simulink model "DKM"  (R2015a)
settings: Solver=ode45  StartTime=0.0  StopTime=10.0  RelTol=1e-3
values from neighbouring files (symbols this model uses):
  L = 0.13    [staticInit.m]
  r = 0.1    [staticInit.m]
settings Model: CovModelRefEnable=off  Creator=Subodh  LastModifiedBy=Subodh
settings DataIOCC: SaveFormat=Dataset
settings HardwareCC: ProdBitPerPointer=64  ProdLargestAtomicFloat=Float  ProdIntDivRoundTo=Zero  ProdEndianess=LittleEndian  ProdHWDeviceType=Specified
settings GRTTargetCC: GeneratePreprocessorConditionals=Use local settings

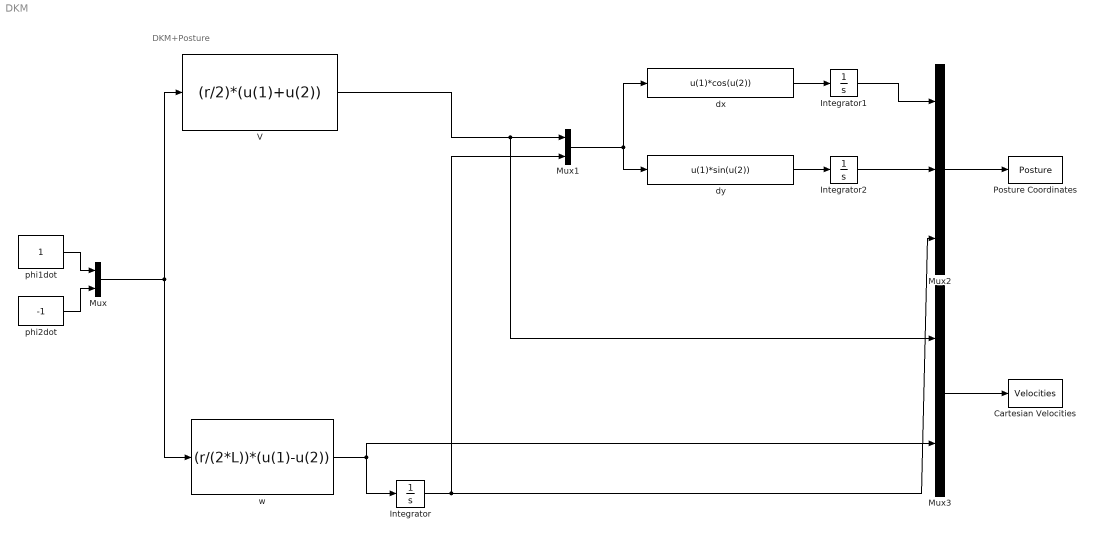
== system DKM ==
  note: DKM+Posture
  Cartesian Velocities : ToWorkspace  VariableName=Velocities  SampleTime=-1
  Integrator : Integrator  InitialCondition=pi
  Integrator1 : Integrator  InitialCondition=2.45
  Integrator2 : Integrator
  Mux : Mux  Inputs=2
  Mux1 : Mux  Inputs=2
  Mux2 : Mux  Inputs=3
  Mux3 : Mux  Inputs=2
  Posture Coordinates : ToWorkspace  VariableName=Posture  SampleTime=-1
  V : Fcn  Expr=(r/2)*(u(1)+u(2))
  dx : Fcn  Expr=u(1)*cos(u(2))
  dy : Fcn  Expr=u(1)*sin(u(2))
  phi1dot : Constant
  phi2dot : Constant  Value=-1
  w : Fcn  Expr=(r/(2*L))*(u(1)-u(2))
  wires:
  phi1dot/1 -> Mux/1
  phi2dot/1 -> Mux/2
  Mux3/1 -> Cartesian Velocities/1
  Mux2/1 -> Posture Coordinates/1
  Integrator2/1 -> Mux2/2
  Integrator1/1 -> Mux2/1
  Integrator/1 -> Mux1/2, Mux2/3
  V/1 -> Mux3/1, Mux1/1
  dx/1 -> Integrator1/1
  Mux1/1 -> dx/1, dy/1
  dy/1 -> Integrator2/1
  w/1 -> Integrator/1, Mux3/2
  Mux/1 -> w/1, V/1
